simulink model "gur_differences"  (R2015b)
settings: Solver=ode45  StartTime=0.0  StopTime=300  RelTol=1e-3
model workspace (MAT data in the model file):
  ODf = 0.01
  gur20151013_24hour : sldodialogs.data.SessionData (value not decoded)
  gur20151013_2hour : sldodialogs.data.SessionData (value not decoded)
  kcat = 4592.3025632
  km = 53768.8232554
settings Model: Creator=sekark  LastModifiedBy=sekark
settings DataIOCC: LimitDataPoints=off  SaveFormat=Array
settings HardwareCC: ProdBitPerPointer=32  ProdLargestAtomicFloat=None  ProdIntDivRoundTo=Undefined  ProdEndianess=Unspecified  ProdWordSize=32  ProdHWDeviceType=32-bit Generic
settings GRTTargetCC: GeneratePreprocessorConditionals=Disable all
settings ConfigComp: CovModelRefEnable=Off

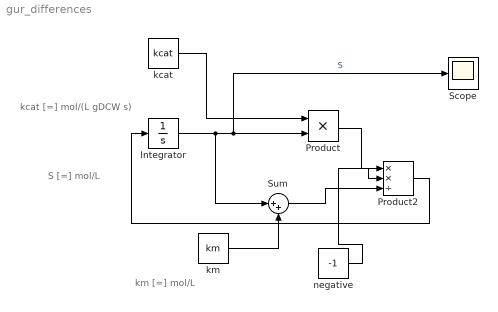
== system gur_differences ==
  note: S [=] mol/L
  note: kcat [=] mol/(L gDCW s)
  note: km [=] mol/L
  Integrator : Integrator  InitialCondition=8000
  Product : Product
  Product2 : Product  Inputs=**/
  Scope : Scope
  Sum : Sum  Inputs=|++
  "kcat " : Constant  Value=kcat
  km : Constant  Value=km
  negative : Constant  Value=-1
  wires:
  Integrator/1 -> Sum/1, Scope/1, Product/2  "S"
  km/1 -> Sum/2
  Product/1 -> Product2/2
  Sum/1 -> Product2/3
  negative/1 -> Product2/1
  Product2/1 -> Integrator/1
  "kcat "/1 -> Product/1
